simulink model "lab341"  (R2023a)
settings: Solver=FixedStepAuto  StartTime=0.0  StopTime=50  FixedStep=0.01  RelTol=1e-3
settings Model: Creator=wendy  LastModifiedBy=wendy

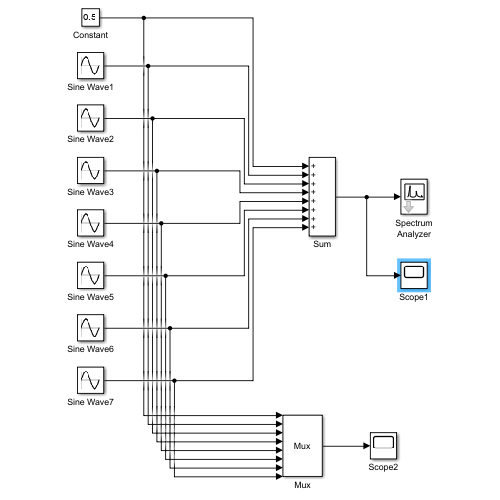
[thumbnail: Simulink's stored preview of the top-level diagram]
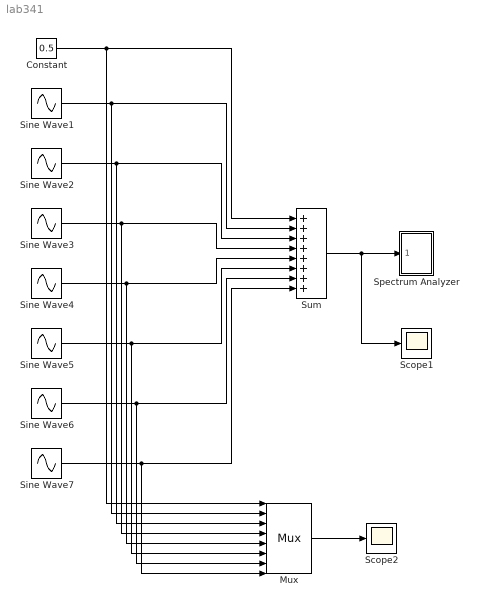
== system lab341 ==
  Constant : Constant  Value=0.5
  Mux : Mux  Inputs=8
  Scope1 : Scope
  Scope2 : Scope
  Sine Wave1 : Sin  Amplitude=2/pi  Frequency=pi  SampleTime=0
  Sine Wave2 : Sin  Amplitude=-2/(3*pi)  Frequency=3*pi  Phase=-pi  SampleTime=0
  Sine Wave3 : Sin  Amplitude=2/(5*pi)  Frequency=5*pi  Phase=-2*pi  SampleTime=0
  Sine Wave4 : Sin  Amplitude=-2/(7*pi)  Frequency=7*pi  Phase=-3*pi  SampleTime=0
  Sine Wave5 : Sin  Amplitude=2/(9*pi)  Frequency=9*pi  Phase=-4*pi  SampleTime=0
  Sine Wave6 : Sin  Amplitude=-2/(11*pi)  Frequency=11*pi  Phase=-5*pi  SampleTime=0
  Sine Wave7 : Sin  Amplitude=2/(13*pi)  Frequency=13*pi  Phase=-6*pi  SampleTime=0
  Spectrum Analyzer : Subsystem  mask(Spectrum analyzer.){N=1024, T_s=0.01, plot_period=10}
      mask prompts: N "Number of sample points:"; T_s "Sampling period (sec):"; plot_period "Plotting Period (sec):"
      mask Help: EE438 Lab utility; See Prof. Bouman.
      mask Display: plot(0,0,100,100,[14,91,91,14,14],[86,86,40,40,86],[85,82,80,79,75,67,63,60,57,53,41,36,33,27,24],[49,50,53,50,49,51,54,66,54,50,50,52,81,51,49])
  Sum : Sum  Inputs=++++++++  InputSameDT=on  SaturateOnIntegerOverflow=on  OutDataTypeStr=Inherit: Same as first input
  wires:
  Sine Wave1/1 -> Mux/2, Sum/2
  Sine Wave2/1 -> Mux/3, Sum/3
  Sine Wave5/1 -> Mux/6, Sum/6
  Sine Wave3/1 -> Mux/4, Sum/4
  Constant/1 -> Mux/1, Sum/1
  Sine Wave4/1 -> Mux/5, Sum/5
  Sine Wave7/1 -> Mux/8, Sum/8
  Mux/1 -> Scope2/1
  Sum/1 -> Scope1/1, Spectrum Analyzer/1(input signal)
  Sine Wave6/1 -> Mux/7, Sum/7

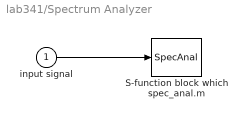
== system lab341/Spectrum Analyzer ==
  input signal : Inport
  S-function block which spec_anal.m : S-Function  FunctionName=SpecAnal  Parameters=N,T_s,plot_period  SFunctionDeploymentMode=off  EnableBusSupport=off
  wires:
  input signal/1 -> S-function block which spec_anal.m/1
